simulink model "LQR"  (R2020b)
settings: Solver=VariableStepAuto  StartTime=0.0  StopTime=2500  RelTol=1e-3
undefined symbols (not defined in the file): A, B, C, Continuous, D, K3, Time, X_0
libraries: ctrlSharedLib x2
settings Model: Creator=kaleb's X1  LastModifiedBy=apulido

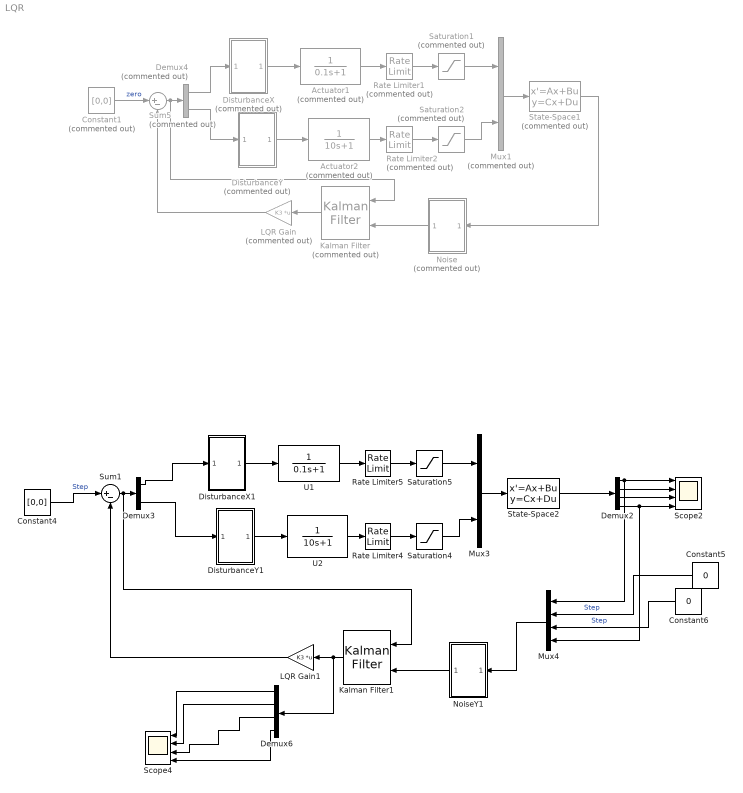
== system LQR ==
  Actuator1 : TransferFcn  Commented=on  Denominator=[0.1 1]
  Actuator2 : TransferFcn  Commented=on  Denominator=[10 1]
  Constant1 : Constant  Commented=on  Value=[0,0]
  Constant4 : Constant  Value=[0,0]
  Constant5 : Constant  Value=0
  Constant6 : Constant  Value=0
  Demux2 : Demux
  Demux3 : Demux  Outputs=2
  Demux4 : Demux  Commented=on  Outputs=2
  Demux6 : Demux
  DisturbanceX : Subsystem  Commented=on
  DisturbanceX1 : Subsystem
  DisturbanceY : Subsystem  Commented=on
  DisturbanceY1 : Subsystem
  Kalman Filter : ctrlSharedLib/Kalman Filter  Commented=on  TimeDomain=Continuous-Time  UseCurrentEstimator=on  ModelSource=Individual A, B, C, D matrices  ModelSourceVariable=ss(0.95,1,1,0,1)  A=A  B=B  C=C  D=D  NumberOfStates=1  NumberOfInputs=1  NumberOfOutputs=1  InitialEstimateSource=Dialog  X0=X_0(1:4)  P0=10  UseK=off  UseGH=off  NumberOfProcessNoiseInputs=1  G=1  TimeInvariantG=on  H=0  TimeInvariantH=on  Q=0.05  TimeInvariantQ=on  R=1  TimeInvariantR=on  N=0  TimeInvariantN=on  AddInputPort=on  AddEnablePort=off  OutputEstimatedY=off  OutputP=off  Ts=-1
  Kalman Filter1 : ctrlSharedLib/Kalman Filter  TimeDomain=Continuous-Time  UseCurrentEstimator=on  ModelSource=Individual A, B, C, D matrices  ModelSourceVariable=ss(0.95,1,1,0,1)  A=A  B=B  C=C  D=D  NumberOfStates=1  NumberOfInputs=1  NumberOfOutputs=1  InitialEstimateSource=Dialog  X0=X_0(1:4)  P0=10  UseK=off  UseGH=off  NumberOfProcessNoiseInputs=1  G=1  TimeInvariantG=on  H=0  TimeInvariantH=on  Q=0.05  TimeInvariantQ=on  R=1  TimeInvariantR=on  N=0  TimeInvariantN=on  AddInputPort=on  AddEnablePort=off  OutputEstimatedY=off  OutputP=off  Ts=-1
  LQR Gain : Gain  Commented=on  Gain=K3  Multiplication=Matrix(K*u)
  LQR Gain1 : Gain  Gain=K3  Multiplication=Matrix(K*u)
  Mux1 : Mux  Commented=on  Inputs=2
  Mux3 : Mux  Inputs=2
  Mux4 : Mux
  Noise : Subsystem  Commented=on
  NoiseY1 : Subsystem
  Rate Limiter1 : RateLimiter  Commented=on  RisingSlewLimit=30  FallingSlewLimit=-30  SampleTimeMode=inherited
  Rate Limiter2 : RateLimiter  Commented=on  RisingSlewLimit=30  FallingSlewLimit=-30  SampleTimeMode=inherited
  Rate Limiter4 : RateLimiter  RisingSlewLimit=30  FallingSlewLimit=-30  SampleTimeMode=inherited
  Rate Limiter5 : RateLimiter  RisingSlewLimit=30  FallingSlewLimit=-30  SampleTimeMode=inherited
  Saturation1 : Saturate  Commented=on  UpperLimit=5880  LowerLimit=-5880
  Saturation2 : Saturate  Commented=on  UpperLimit=5880  LowerLimit=-5880
  Saturation4 : Saturate  UpperLimit=5880  LowerLimit=-5880
  Saturation5 : Saturate  UpperLimit=5880  LowerLimit=-5880
  Scope2 : Scope  NumInputPorts=4
  Scope4 : Scope  NumInputPorts=4
  State-Space1 : StateSpace  Commented=on  A=A  B=B  C=C  D=D  InitialCondition=[-3.10; -39.16; 0.00002; 0.0041]
  State-Space2 : StateSpace  A=A  B=B  C=C  D=D  InitialCondition=[-3.10; -39.16; 0.00002; 0.0041]
  Sum1 : Sum  Inputs=|+-
  Sum5 : Sum  Commented=on  Inputs=|+-
  U1 : TransferFcn  Denominator=[0.1 1]
  U2 : TransferFcn  Denominator=[10 1]
  wires:
  Constant1/1 -> Sum5/1  "zero"
  Mux1/1 -> State-Space1/1
  Actuator2/1 -> Rate Limiter2/1
  Rate Limiter1/1 -> Saturation1/1
  Actuator1/1 -> Rate Limiter1/1
  Saturation1/1 -> Mux1/1
  Rate Limiter2/1 -> Saturation2/1
  Saturation2/1 -> Mux1/2
  Demux4/1 -> DisturbanceX/1(In1)
  Demux4/2 -> DisturbanceY/1(In1)
  Sum5/1 -> Kalman Filter/1, Demux4/1
  LQR Gain/1 -> Sum5/2
  Kalman Filter/1 -> LQR Gain/1
  Noise/1(Out1) -> Kalman Filter/2
  State-Space1/1 -> Noise/1(In1)
  DisturbanceX/1(Out1) -> Actuator1/1
  DisturbanceY/1(Out1) -> Actuator2/1
  Saturation4/1 -> Mux3/2
  Demux2/1 -> Scope2/1, Mux4/1
  Constant5/1 -> Mux4/2  "Step"
  LQR Gain1/1 -> Sum1/2
  Mux4/1 -> NoiseY1/1(In1)
  Constant6/1 -> Mux4/3  "Step"
  State-Space2/1 -> Demux2/1
  DisturbanceY1/1(Out1) -> U2/1
  Demux2/3 -> Scope2/3
  Rate Limiter5/1 -> Saturation5/1
  NoiseY1/1(Out1) -> Kalman Filter1/2
  Demux6/2 -> Scope4/2
  U1/1 -> Rate Limiter5/1
  Demux3/2 -> DisturbanceY1/1(In1)
  Sum1/1 -> Kalman Filter1/1, Demux3/1
  Kalman Filter1/1 -> Demux6/1, LQR Gain1/1
  Demux6/3 -> Scope4/3
  Demux3/1 -> DisturbanceX1/1(In1)
  Demux6/4 -> Scope4/4
  Rate Limiter4/1 -> Saturation4/1
  U2/1 -> Rate Limiter4/1
  DisturbanceX1/1(Out1) -> U1/1
  Saturation5/1 -> Mux3/1
  Constant4/1 -> Sum1/1  "Step"
  Mux3/1 -> State-Space2/1
  Demux2/2 -> Scope2/2
  Demux6/1 -> Scope4/1
  Demux2/4 -> Mux4/4, Scope2/4

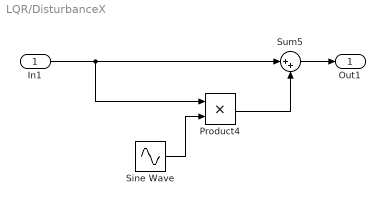
== system LQR/DisturbanceX ==
  In1 : Inport
  Product4 : Product
  Sine Wave : Sin  Amplitude=0.03  SampleTime=0
  Sum5 : Sum  Inputs=|++
  Out1 : Outport
  wires:
  In1/1 -> Product4/1, Sum5/1
  Product4/1 -> Sum5/2
  Sine Wave/1 -> Product4/2
  Sum5/1 -> Out1/1

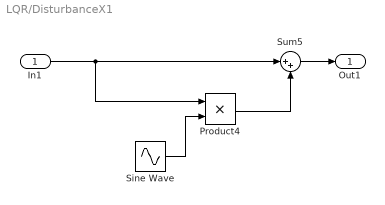
== system LQR/DisturbanceX1 ==
  In1 : Inport
  Product4 : Product
  Sine Wave : Sin  Amplitude=0.03  SampleTime=0
  Sum5 : Sum  Inputs=|++
  Out1 : Outport
  wires:
  In1/1 -> Product4/1, Sum5/1
  Product4/1 -> Sum5/2
  Sine Wave/1 -> Product4/2
  Sum5/1 -> Out1/1

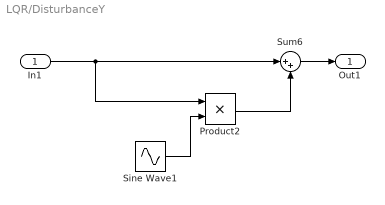
== system LQR/DisturbanceY ==
  In1 : Inport
  Product2 : Product
  Sine Wave1 : Sin  Amplitude=0.03  SampleTime=0
  Sum6 : Sum  Inputs=|++
  Out1 : Outport
  wires:
  Product2/1 -> Sum6/2
  In1/1 -> Product2/1, Sum6/1
  Sine Wave1/1 -> Product2/2
  Sum6/1 -> Out1/1

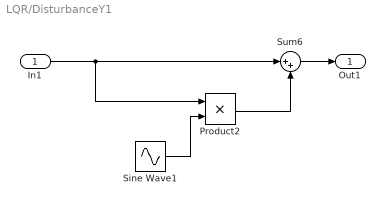
== system LQR/DisturbanceY1 ==
  In1 : Inport
  Product2 : Product
  Sine Wave1 : Sin  Amplitude=0.03  SampleTime=0
  Sum6 : Sum  Inputs=|++
  Out1 : Outport
  wires:
  Product2/1 -> Sum6/2
  In1/1 -> Product2/1, Sum6/1
  Sine Wave1/1 -> Product2/2
  Sum6/1 -> Out1/1

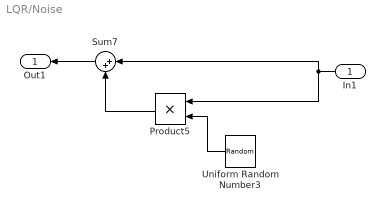
== system LQR/Noise ==
  In1 : Inport
  Product5 : Product
  Sum7 : Sum  Inputs=|++
  Uniform Random Number3 : UniformRandomNumber  Minimum=-0.08  Maximum=0.08  SampleTime=0.01
  Out1 : Outport
  wires:
  Uniform Random Number3/1 -> Product5/2
  In1/1 -> Product5/1, Sum7/1
  Product5/1 -> Sum7/2
  Sum7/1 -> Out1/1

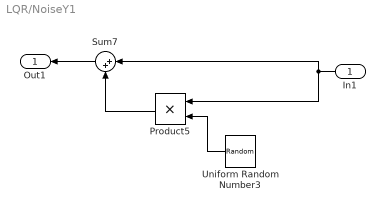
== system LQR/NoiseY1 ==
  In1 : Inport
  Product5 : Product
  Sum7 : Sum  Inputs=|++
  Uniform Random Number3 : UniformRandomNumber  Minimum=-0.08  Maximum=0.08  SampleTime=0.01
  Out1 : Outport
  wires:
  Uniform Random Number3/1 -> Product5/2
  In1/1 -> Product5/1, Sum7/1
  Product5/1 -> Sum7/2
  Sum7/1 -> Out1/1
